simulink model "Part7_Creating_2D_Traffic_Visualization"  (R2021a)
settings: Solver=VariableStepAuto  StartTime=0.0  StopTime=30  RelTol=1e-3
libraries: vrlib x2, simulink x1, mpcadaslib x1
settings Model: Creator=QZHAN112  LastModifiedBy=QZHAN112

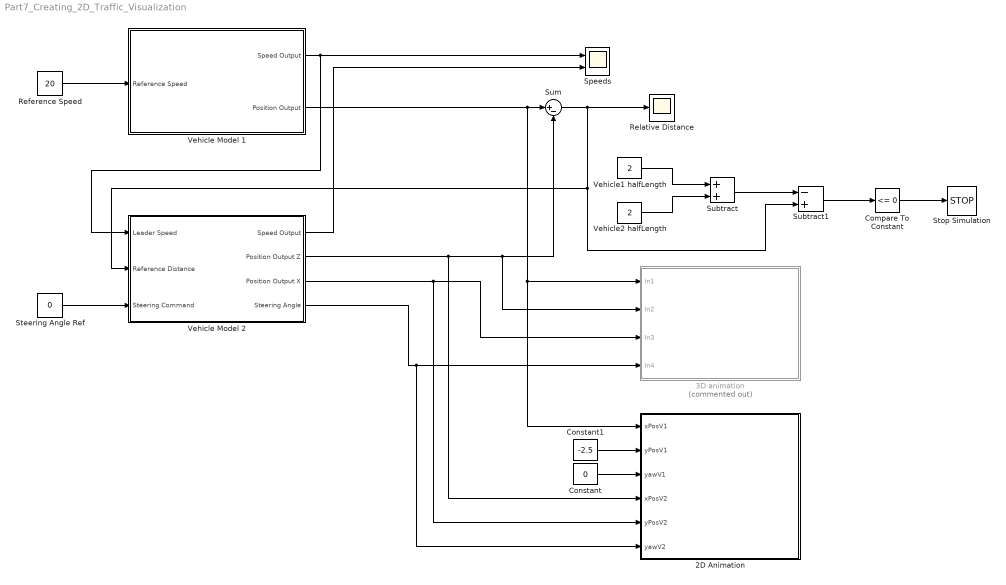
== system Part7_Creating_2D_Traffic_Visualization ==
  2D Animation : Subsystem
  3D animation : Subsystem  Commented=on
  Compare To Constant : simulink/Logic and Bit Operations/Compare To Constant  relop=<=  const=0  OutDataTypeStr=boolean
  Constant : Constant  Value=0
  Constant1 : Constant  Value=-2.5
  Reference Speed : Constant  Value=20
  Relative Distance : Scope
  Speeds : Scope  NumInputPorts=2
  Steering Angle Ref : Constant  Value=0
  Stop Simulation : Stop
  Subtract : Sum
  Subtract1 : Sum  Inputs=-+
  Sum : Sum  Inputs=|+-
  Vehicle Model 1 : Subsystem  mask{Pos=10, Speed=15}
      mask prompts: Pos "Initial Position"; Speed "Initial Speed"
      mask TypeOptions Pos: Initial Position/Value
      mask TypeOptions Speed: Initial Speed/Value
      mask Display: image('model-based autonomous traffic simulation framework\Scratch.jpg');
  Vehicle Model 2 : Subsystem  mask{Pos=0, Speed=30}
      mask prompts: Pos "Initial Position"; Speed "Initial Speed"
      mask TypeOptions Pos: Initial Position Z/Value
      mask TypeOptions Speed: Initial Speed/Value
      mask Display: image('model-based autonomous traffic simulation framework\Car-Design-Drawing-From-Shoulder.jpg');
  Vehicle1 halfLength : Constant  Value=2
  Vehicle2 halfLength : Constant  Value=2
  wires:
  Vehicle Model 1/2(Position Output) -> 2D Animation/1(xPosV1), 3D animation/1(In1), Sum/1
  Reference Speed/1 -> Vehicle Model 1/1(Reference Speed)
  Vehicle Model 2/1(Speed Output) -> Speeds/2
  Vehicle Model 1/1(Speed Output) -> Speeds/1, Vehicle Model 2/1(Leader Speed)
  Sum/1 -> Relative Distance/1, Vehicle Model 2/2(Reference Distance), Subtract1/2
  Vehicle Model 2/2(Position Output Z) -> 2D Animation/4(xPosV2), Sum/2, 3D animation/2(In2)
  Compare To Constant/1 -> Stop Simulation/1
  Steering Angle Ref/1 -> Vehicle Model 2/3(Steering Command)
  Vehicle Model 2/3(Position Output X) -> 2D Animation/5(yPosV2), 3D animation/3(In3)
  Vehicle Model 2/4(Steering Angle) -> 2D Animation/6(yawV2), 3D animation/4(In4)
  Constant/1 -> 2D Animation/3(yawV1)
  Constant1/1 -> 2D Animation/2(yPosV1)
  Vehicle1 halfLength/1 -> Subtract/1
  Vehicle2 halfLength/1 -> Subtract/2
  Subtract/1 -> Subtract1/1
  Subtract1/1 -> Compare To Constant/1

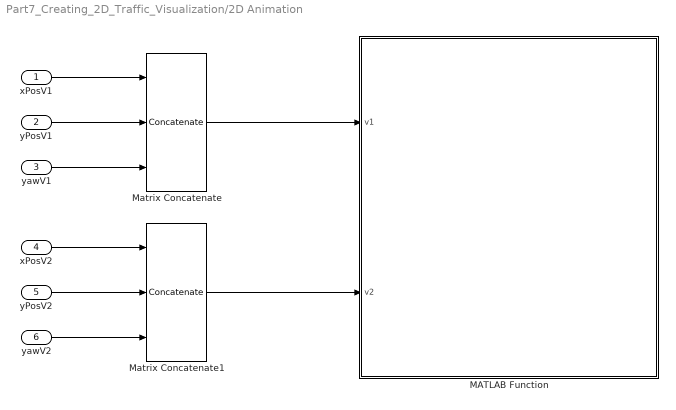
== system Part7_Creating_2D_Traffic_Visualization/2D Animation ==
  xPosV1 : Inport
  yPosV1 : Inport  Port=2
  yawV1 : Inport  Port=3
  xPosV2 : Inport  Port=4
  yPosV2 : Inport  Port=5
  yawV2 : Inport  Port=6
  MATLAB Function : MATLAB Function  TreatAsAtomicUnit=on
      mask init:
      | close all;
      | figure('units','normalized','outerposition',[0 0 1 1]);
      | % grid on
      | axis equal;
      | hold on
  Matrix Concatenate : Concatenate  NumInputs=3  ConcatenateDimension=2
  Matrix Concatenate1 : Concatenate  NumInputs=3  ConcatenateDimension=2
  wires:
  Matrix Concatenate/1 -> MATLAB Function/1(v1)
  yawV1/1 -> Matrix Concatenate/3
  yPosV1/1 -> Matrix Concatenate/2
  xPosV1/1 -> Matrix Concatenate/1
  xPosV2/1 -> Matrix Concatenate1/1
  yPosV2/1 -> Matrix Concatenate1/2
  yawV2/1 -> Matrix Concatenate1/3
  Matrix Concatenate1/1 -> MATLAB Function/2(v2)

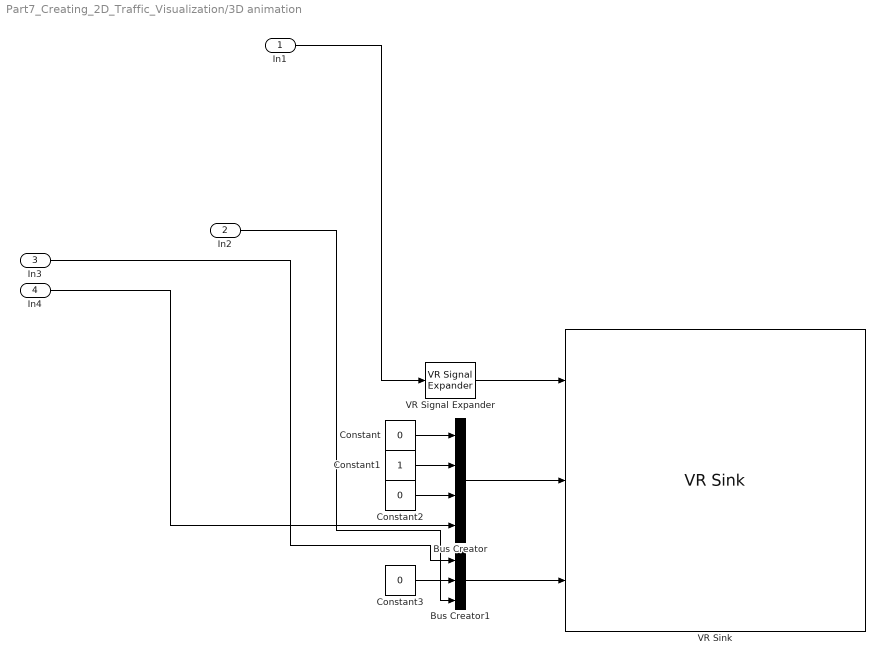
== system Part7_Creating_2D_Traffic_Visualization/3D animation ==
  In1 : Inport
  In2 : Inport  Port=2
  In3 : Inport  Port=3
  In4 : Inport  Port=4
  Bus Creator : BusCreator  Inputs=4
  Bus Creator1 : BusCreator  Inputs=3
  Constant : Constant  Value=0
  Constant1 : Constant
  Constant2 : Constant  Value=0
  Constant3 : Constant  Value=0
  VR Signal Expander : vrlib/VR Signal Expander  outwidth=3  outidx=[3]
  VR Sink : vrlib/VR Sink  InstantiateOnLoad=on  SampleTime=0.05  ViewEnable=on  RemoteChange=off  RemoteView=off  FieldsWritten=Car_Red.translation.3.1.1.double#Car_Blue.rotation.4.1.1.double#Car_Blue.translation.3.1.1.double  WorldFileName=PlatoonWorld.WRL  AutoView=off  VideoDimensions=[]  AllowVariableSize=off
  wires:
  Bus Creator1/1 -> VR Sink/3
  Constant1/1 -> Bus Creator/2
  VR Signal Expander/1 -> VR Sink/1
  Constant2/1 -> Bus Creator/3
  Constant/1 -> Bus Creator/1
  Bus Creator/1 -> VR Sink/2
  Constant3/1 -> Bus Creator1/2
  In3/1 -> Bus Creator1/1
  In4/1 -> Bus Creator/4
  In1/1 -> VR Signal Expander/1
  In2/1 -> Bus Creator1/3

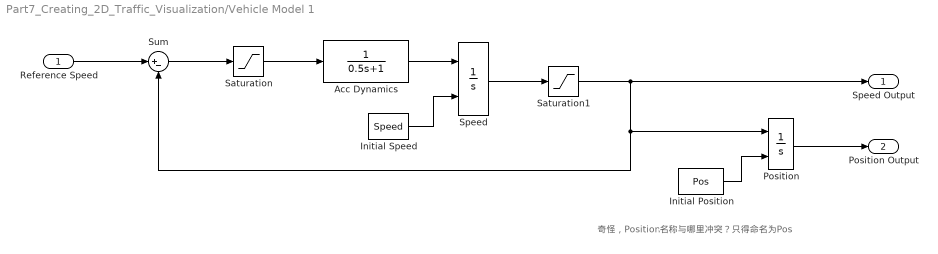
== system Part7_Creating_2D_Traffic_Visualization/Vehicle Model 1 ==
  note: 奇怪，Position名称与哪里冲突？只得命名为Pos
  Reference Speed : Inport
  Acc Dynamics : TransferFcn  Denominator=[0.5 1]
  Initial Position : Constant  Value=Pos
  Initial Speed : Constant  Value=Speed
  Position : Integrator  InitialConditionSource=external
  Saturation : Saturate  UpperLimit=2  LowerLimit=-3
  Saturation1 : Saturate  UpperLimit=inf  LowerLimit=0
  Speed : Integrator  InitialConditionSource=external
  Sum : Sum  Inputs=|+-
  Speed Output : Outport
  Position Output : Outport  Port=2
  wires:
  Saturation/1 -> Acc Dynamics/1
  Acc Dynamics/1 -> Speed/1
  Speed/1 -> Saturation1/1
  Position/1 -> Position Output/1
  Saturation1/1 -> Speed Output/1, Sum/2, Position/1
  Reference Speed/1 -> Sum/1
  Initial Speed/1 -> Speed/2
  Sum/1 -> Saturation/1
  Initial Position/1 -> Position/2

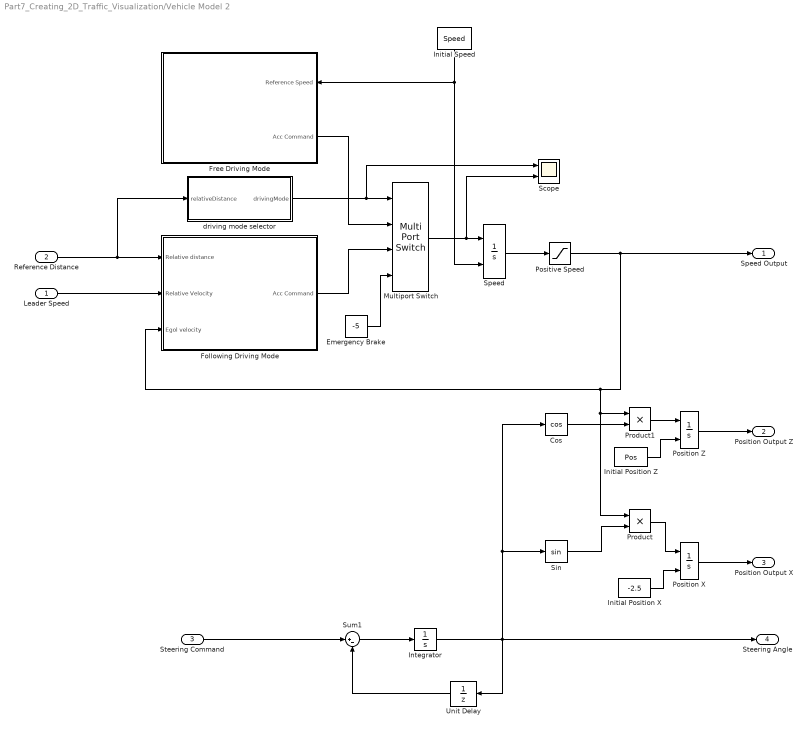
== system Part7_Creating_2D_Traffic_Visualization/Vehicle Model 2 ==
  Leader Speed : Inport
  Reference Distance : Inport  Port=2
  Steering Command : Inport  Port=3
  Cos : Trigonometry  Operator=cos
  Emergency Brake : Constant  Value=-5
  Following Driving Mode : Subsystem
  Free Driving Mode : Subsystem
      settings: PortSchema="{\"entries\":[{\"content\":{\"sides\":[{\"content\":{\"connectorIds\":[]},\"type\":\"ConnectorPlacement.EquallySpacedRectSide\",\"uuid\":\"610b25c5-b833-48d8-91de-4e4522f1e869\"},{\"content\":{\"connectorIds\":[\"In1\",\"Out1\"],\"side\":\"RIGHT\"},\"type\":\"ConnectorPlacement.EquallySpacedRectSide\",\"uuid\":\"bfbfafdf-9638-4c83-9a6c-a30c0fb24eff\"},{\"content\":{\"connectorIds\":[],\"side\":\"TOP\"},\"type\":\"ConnectorPlacement.EquallySpacedRectSide\",\"uuid\":\"2708cd9c-977e-4237-a5bd-2827f533dc12\"}]},\"type\":\"ConnectorPlacement.EquallySpacedConnector\",\"uuid\":\"23ea83fe-0fb5-46b9-9450-330af3b093f3\"}],\"packageUris\":[\"http://schema.mathworks.com/mf0/Connector/R2020b\"],\"version\":\"1.0\"}"
  Initial Position X : Constant  Value=-2.5
  Initial Position Z : Constant  Value=Pos
  Initial Speed : Constant  Value=Speed
  Integrator : Integrator
  Multiport Switch : MultiPortSwitch
  Position X : Integrator  InitialConditionSource=external
  Position Z : Integrator  InitialConditionSource=external
  Positive Speed : Saturate  UpperLimit=inf  LowerLimit=0
  Product : Product
  Product1 : Product
  Scope : Scope  NumInputPorts=2
  Sin : Trigonometry
  Speed : Integrator  InitialConditionSource=external
  Sum1 : Sum  Inputs=|+-
  Unit Delay : UnitDelay  SampleTime=-1  HasFrameUpgradeWarning=on
  driving mode selector : Stateflow chart  TreatAsAtomicUnit=on
  Speed Output : Outport
  Position Output Z : Outport  Port=2
  Position Output X : Outport  Port=3
  Steering Angle : Outport  Port=4
  wires:
  Speed/1 -> Positive Speed/1
  Position Z/1 -> Position Output Z/1
  Initial Speed/1 -> Speed/2, Free Driving Mode/1(Reference Speed)
  Initial Position Z/1 -> Position Z/2
  Positive Speed/1 -> Speed Output/1, Following Driving Mode/3(Egol velocity), Product/1, Product1/1
  Sum1/1 -> Integrator/1
  Steering Command/1 -> Sum1/1
  Integrator/1 -> Steering Angle/1, Cos/1, Sin/1, Unit Delay/1
  Unit Delay/1 -> Sum1/2
  Sin/1 -> Product/2
  Initial Position X/1 -> Position X/2
  Position X/1 -> Position Output X/1
  Product/1 -> Position X/1
  Cos/1 -> Product1/2
  Product1/1 -> Position Z/1
  Reference Distance/1 -> driving mode selector/1(relativeDistance), Following Driving Mode/1(Relative distance)
  Leader Speed/1 -> Following Driving Mode/2(Relative Velocity)
  Following Driving Mode/1(Acc Command) -> Multiport Switch/3
  Free Driving Mode/1(Acc Command) -> Multiport Switch/2
  Multiport Switch/1 -> Scope/2, Speed/1
  Emergency Brake/1 -> Multiport Switch/4
  driving mode selector/1(drivingMode) -> Scope/1, Multiport Switch/1

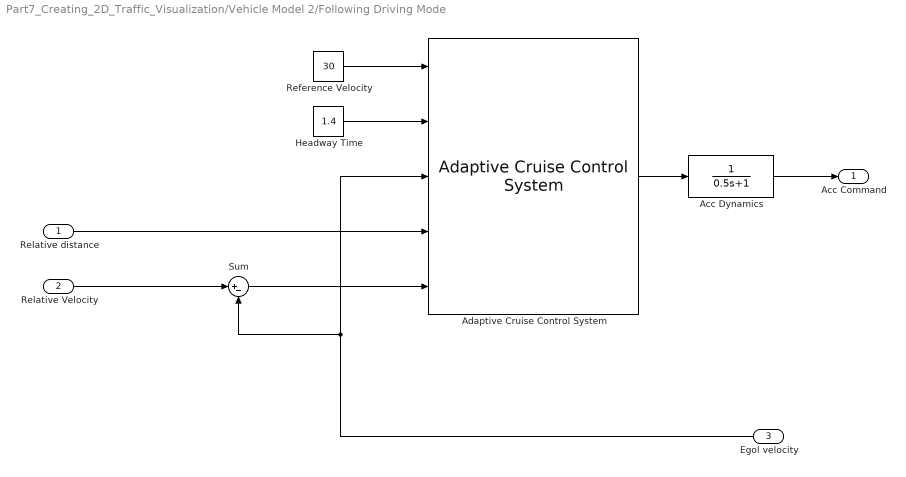
== system Part7_Creating_2D_Traffic_Visualization/Vehicle Model 2/Following Driving Mode ==
  Relative distance : Inport
  Relative Velocity : Inport  Port=2
  Egol velocity : Inport  Port=3
  Acc Dynamics : TransferFcn  Denominator=[0.5 1]
  Adaptive Cruise Control System : mpcadaslib/Adaptive Cruise Control System  EgoModel=tf(1,[0.5,1,0])  InitialEgoVelocity=30  DefaultSpacing=10  MaxVelocity=50  MinAcceleration=-3  amin_ext=off  MaxAcceleration=2  amax_ext=off  Ts=0.1  PredictionHorizon=300  ControllerBehavior=0.800  suboptimal=off  maxiter=10  datatypeopt=double  optmode=off  trackmode=off
  Headway Time : Constant  Value=1.4
  Reference Velocity : Constant  Value=30
  Sum : Sum  Inputs=|+-
  Acc Command : Outport
  wires:
  Adaptive Cruise Control System/1 -> Acc Dynamics/1
  Sum/1 -> Adaptive Cruise Control System/5
  Reference Velocity/1 -> Adaptive Cruise Control System/1
  Relative distance/1 -> Adaptive Cruise Control System/4
  Egol velocity/1 -> Adaptive Cruise Control System/3, Sum/2
  Relative Velocity/1 -> Sum/1
  Headway Time/1 -> Adaptive Cruise Control System/2
  Acc Dynamics/1 -> Acc Command/1

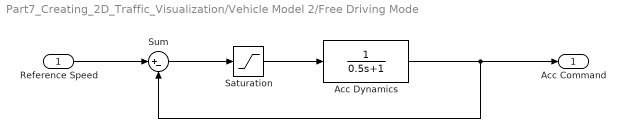
== system Part7_Creating_2D_Traffic_Visualization/Vehicle Model 2/Free Driving Mode ==
  Reference Speed : Inport
  Acc Dynamics : TransferFcn  Denominator=[0.5 1]
  Saturation : Saturate  UpperLimit=2  LowerLimit=-3
  Sum : Sum  Inputs=|+-
  Acc Command : Outport
  wires:
  Saturation/1 -> Acc Dynamics/1
  Acc Dynamics/1 -> Sum/2, Acc Command/1
  Sum/1 -> Saturation/1
  Reference Speed/1 -> Sum/1

== stateflow chart Part7_Creating_2D_Traffic_Visualization/Vehicle Model 2/driving mode selector ==
  state FollowingMode
    entry:
    drivingMode = 2;
  state FreeMode
    entry:
    drivingMode = 1;
  state EmergencyBrake
    entry:
    drivingMode = 3;
  (default) -> FreeMode
  FollowingMode -> FreeMode [order 1] : [relativeDistance > 60]
  FreeMode -> FollowingMode [order 1] : [relativeDistance <= 50]
  FreeMode -> EmergencyBrake [order 2] : [relativeDistance <= 25]
  FollowingMode -> EmergencyBrake [order 2] : [relativeDistance <= 25]
  EmergencyBrake -> FollowingMode : [relativeDistance >= 30]
  data: drivingMode output; relativeDistance input

== matlab function Part7_Creating_2D_Traffic_Visualization/2D Animation/MATLAB Function ==
  data: v1 input; v2 input
function plotVehicle(v1, v2)

% Clear previous vehicle
cla;

for v=[v1, v2]

    x = v(1);
    y = v(2);
    yaw = v(3);

    centerP = [x; y];
    halflength_v = 2;
    halfwidth_v = 1;

    % Create a retangle represent a vehicle
    p1 = [ halflength_v;  halfwidth_v];
    p2 = [ halflength_v; -halfwidth_v];
    p3 = [-halflength_v; -halfwidth_v];
    p4 = [-halflength_v;  halfwidth_v];

    % Rotation Matrix
    rotatrix = [cos(yaw) -sin(yaw); sin(yaw) cos(yaw)];

    % Rotated Points
    % 这里用极坐标的参数方程来推导，然后用矩阵和向量的乘法
    % x = rcosθ     
    % y = rsinθ
    % x' = rcos(θ + A) => r(cosθcosA - sinθsinA) => rcosθcosA - rsinθsinA
    %                                            => xcosA - ysinA
    % y' = rsin(θ + A) => r(sinθcosA + cosθsinA) => rsinθcosA + rcosθsinA
    %                                            => ycosA + xsinA
    % 
    % |cosA -sinA| |x|       |xcosA - ysinA|
    % |sinA  cosA| |y|   =>  |xsinA + ycosA|
    %
    p1r = centerP + rotatrix*p1;
    p2r = centerP + rotatrix*p2;
    p3r = centerP + rotatrix*p3;
    p4r = centerP + rotatrix*p4;

    
    % Connecting points
    Hitbox = [p1r p2r p3r p4r p1r];


    % 将5个点的x坐标转化为一个列向量，y也一样
    cornersV_x = transpose(Hitbox(1,:));
    cornersV_y = transpose(Hitbox(2,:));
    
    
    % Plot vehicles
    if v == v1
        plot(cornersV_x,cornersV_y,'b'); % vehicel rectangle
        plot(x,y,'o'); % vehicle center
    else
        plot(cornersV_x,cornersV_y);
        plot(x,y);
    end
    
end


% Plot road
upperline = plot([0 1000],[5 5],'color','#b0c4de','linewidth',4);
midLine = plot([0 1000],[0 0],'--','color','#b0c4de','linewidth',2);
lowerLine = plot([0 1000],[-5 -5],'color','#b0c4de','linewidth',4);


% Adjust axis
axis([x-50 x+50 y-10 y+10]);
